simulink model "MotorXploer_1"  (R2025a)
settings: Solver=FixedStepAuto  StartTime=0.0  StopTime=inf  FixedStep=0.001  RelTol=1e-3
undefined symbols (not defined in the file or in its folder): Blocking, LF, Non
libraries: dspstat3 x4, amg_usbconverter_n_connect_lib x3, dspfdesign x1
settings Model: Creator=beamk  LastModifiedBy=tongl

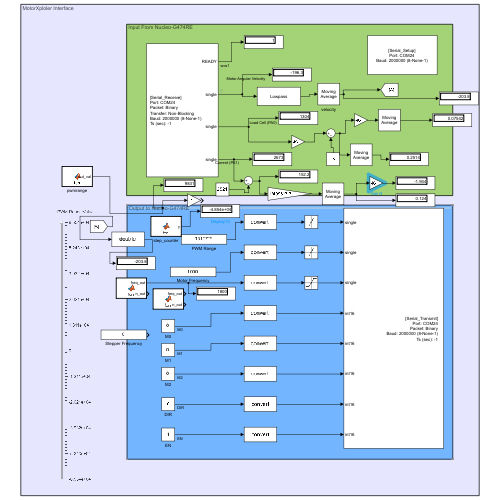
[thumbnail: Simulink's stored preview of the top-level diagram]
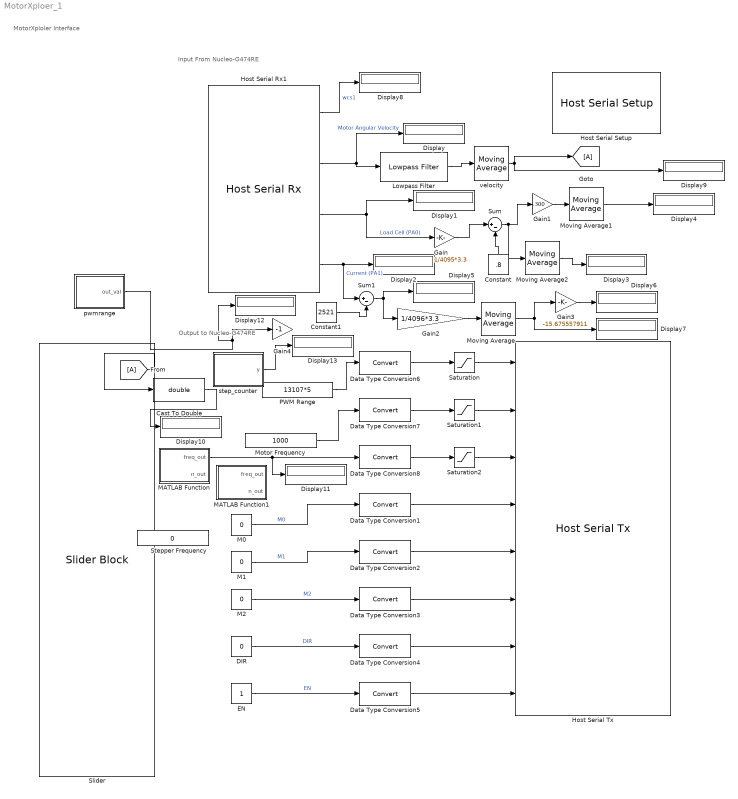
== system MotorXploer_1 ==
  note: Output to Nucleo-G474RE
  note: Input From Nucleo-G474RE
  note: MotorXploler Interface
  Cast To Double : DataTypeConversion  OutDataTypeStr=double  SaturateOnIntegerOverflow=off  RndMeth=Floor
  Constant : Constant  Value=.8
  Constant1 : Constant  Value=2521
  DIR : Constant  Value=0
  Data Type Conversion{1..8} (8 alike) : DataTypeConversion  SaturateOnIntegerOverflow=off  RndMeth=Floor
  Display{,1..13} (14 alike) : Display
  EN : Constant
  From : From
  Gain : Gain  Gain=1/4095*3.3
  Gain1 : Gain  Gain=.300
  Gain2 : Gain  Gain=1/4096*3.3
  Gain3 : Gain  Gain=-15.675557911
  Gain4 : Gain  Gain=-1
  Goto : Goto
  Host Serial Rx1 : amg_usbconverter_n_connect_lib/Host Serial Rx  conf=rx  port=<auto>  baudrate=2000000  databits=8  parity=None  stopbit=1  flowcontrol=None  transfer=Non-Blocking  timeout=5  packetmode=Binary  enableinitialvalues=off  initialvalues=[]  binheader='25'  binterminator='4E'  porttype_double=0  porttype_single=3  porttype_int8=0  porttype_uint8=0  porttype_int16=0  porttype_uint16=0  porttype_int32=0  porttype_uint32=0  asciiformat='%f,%f,%d,%d'  rx_asciiterminator="LF (0x0A - \"\\n\")"  tx_asciiterminator="CRLF (0x0D 0x0A - \"\\r\\n\")"  sampletime=-1  enablecustomportlabel=off  cinputportlabel=0  coutputportlabel=A  portpinstr=0  blockid=HostSerialRx1  inputporttype=[]  inputportwidth=[]  inputportlabel={}  outputporttype=[3 1 1 1]  outputportwidth=[1 1 1 1]  outputportlabel={'READY','single','single','single'}  compat=0  optionstring=[]  autoport='COM24'
  Host Serial Setup : amg_usbconverter_n_connect_lib/Host Serial Setup  conf=setup  port=<auto>  baudrate=2000000  databits=8  parity=None  stopbit=1  flowcontrol=None  transfer=Blocking  timeout=2  packetmode=Binary  initialvalues=[]  binheader='7E 7E'  binterminator='03 03'  porttype_double=0  porttype_single=1  porttype_int8=0  porttype_uint8=0  porttype_int16=0  porttype_uint16=0  porttype_int32=0  porttype_uint32=2  asciiformat='%d %u %x'  rx_asciiterminator="CRLF (0x0D 0x0A - \"\\r\\n\")"  tx_asciiterminator="CRLF (0x0D 0x0A - \"\\r\\n\")"  sampletime=-1  enablecustomportlabel=off  cinputportlabel=0  coutputportlabel=A  portpinstr=0  blockid=HostSerialSetup  inputporttype=[]  inputportwidth=[]  inputportlabel={}  outputporttype=[]  outputportwidth=[]  outputportlabel={}  compat=0  optionstring=[]  autoport='COM24'
  Host Serial Tx : amg_usbconverter_n_connect_lib/Host Serial Tx  conf=tx  port=<auto>  baudrate=2000000  databits=8  parity=None  stopbit=1  flowcontrol=None  transfer=Blocking  timeout=2  packetmode=Binary  initialvalues=[]  binheader='25'  binterminator='4E'  porttype_double=0  porttype_single=3  porttype_int8=0  porttype_uint8=0  porttype_int16=5  porttype_uint16=0  porttype_int32=0  porttype_uint32=0  asciiformat='%d,%f'  rx_asciiterminator="CRLF (0x0D 0x0A - \"\\r\\n\")"  tx_asciiterminator="CRLF (0x0D 0x0A - \"\\r\\n\")"  sampletime=-1  enablecustomportlabel=off  cinputportlabel=0  coutputportlabel=A  portpinstr=0  blockid=HostSerialTx  inputporttype=[1 1 1 4 4 4 4 4]  inputportwidth=[1 1 1 1 1 1 1 1]  inputportlabel={'single','single','single','int16','int16','int16','int16','int16'}  outputporttype=[]  outputportwidth=[]  outputportlabel={}  compat=0  optionstring=[]  autoport='COM24'
      settings: SourceProductName=aMG USB Converter N
  Lowpass Filter : dspfdesign/Lowpass Filter  FilterType=FIR  DesignForMinimumOrder=on  FilterOrder=50  PassbandFrequency=.6  StopbandFrequency=.7  PassbandRipple=0.1  StopbandAttenuation=80  SampleRateMode=Specify on dialog  SampleRate=100  SimulateUsing=Interpreted execution  roundingMode=Floor  coeffsDataTypeStr=fixdt(1,16)
  M0 : Constant  Value=0
  M1 : Constant  Value=0
  M2 : Constant  Value=0
  MATLAB Function : MATLAB Function  TreatAsAtomicUnit=on
  MATLAB Function1 : MATLAB Function  TreatAsAtomicUnit=on
  Motor Frequency : Constant  Value=1000  OutDataTypeStr=single
  Moving Average : dspstat3/Moving Average  Method=Sliding window  ForgettingFactorPort=off  SpecifyWindowLength=on  WindowLength=100  OverlapLength=99  AllowArbitraryInputLength=off  ForgettingFactor=0.9  SimulateUsing=Interpreted execution
  Moving Average1 : dspstat3/Moving Average  Method=Sliding window  ForgettingFactorPort=off  SpecifyWindowLength=on  WindowLength=100  OverlapLength=99  AllowArbitraryInputLength=off  ForgettingFactor=0.9  SimulateUsing=Interpreted execution
  Moving Average2 : dspstat3/Moving Average  Method=Sliding window  ForgettingFactorPort=off  SpecifyWindowLength=on  WindowLength=100  OverlapLength=99  AllowArbitraryInputLength=off  ForgettingFactor=0.9  SimulateUsing=Interpreted execution
  PWM Range : Constant  Value=13107*5  OutDataTypeStr=single
  Saturation : Saturate  UpperLimit=65535  LowerLimit=-65535
  Saturation1 : Saturate  UpperLimit=20000  LowerLimit=0
  Saturation2 : Saturate  UpperLimit=inf  LowerLimit=0
  Slider : SliderBlock  ScaleMin=-65535  ScaleMax=65535
  Stepper Frequency : Constant  Value=0  OutDataTypeStr=single
  Sum : Sum  Inputs=|+-
  Sum1 : Sum  Inputs=|+-
  pwmrange : MATLAB Function  TreatAsAtomicUnit=on
  step_counter : MATLAB Function  TreatAsAtomicUnit=on
  velocity : dspstat3/Moving Average  Method=Sliding window  ForgettingFactorPort=off  SpecifyWindowLength=on  WindowLength=4  OverlapLength=3  AllowArbitraryInputLength=off  ForgettingFactor=0.9  SimulateUsing=Interpreted execution
  wires:
  Host Serial Rx1/2 -> Lowpass Filter/1, Display/1  "Motor Angular Velocity"
  Host Serial Rx1/3 -> Gain/1, Display1/1  "Load Cell (PA0)"
  M0/1 -> Data Type Conversion1/1  "M0"
  EN/1 -> Data Type Conversion5/1  "EN"
  DIR/1 -> Data Type Conversion4/1  "DIR"
  M1/1 -> Data Type Conversion2/1  "M1"
  M2/1 -> Data Type Conversion3/1  "M2"
  Data Type Conversion1/1 -> Host Serial Tx/4
  Data Type Conversion2/1 -> Host Serial Tx/5
  Data Type Conversion3/1 -> Host Serial Tx/6
  Data Type Conversion4/1 -> Host Serial Tx/7
  Data Type Conversion5/1 -> Host Serial Tx/8
  Data Type Conversion6/1 -> Saturation/1
  Saturation/1 -> Host Serial Tx/1
  Data Type Conversion7/1 -> Saturation1/1
  Data Type Conversion8/1 -> Saturation2/1
  Saturation1/1 -> Host Serial Tx/2
  Saturation2/1 -> Host Serial Tx/3
  Host Serial Rx1/4 -> Display2/1, Sum1/1  "Current (PA1)"
  Gain/1 -> Sum/1
  Moving Average2/1 -> Display3/1
  Gain1/1 -> Moving Average1/1
  Sum/1 -> Moving Average2/1, Gain1/1
  Constant/1 -> Sum/2
  Moving Average1/1 -> Display4/1
  Constant1/1 -> Sum1/2
  Sum1/1 -> Gain2/1, Display5/1
  Gain3/1 -> Display6/1
  Moving Average/1 -> Gain3/1, Display7/1
  Gain2/1 -> Moving Average/1
  Host Serial Rx1/1 -> Display8/1  "wcs1"
  Lowpass Filter/1 -> velocity/1
  velocity/1 -> Goto/1, Display9/1
  MATLAB Function/1(freq_out) -> Data Type Conversion8/1, Display11/1
  From/1 -> Cast To Double/1
  Cast To Double/1 -> Display10/1
  pwmrange/1(out_val) -> Display12/1, Gain4/1
  step_counter/1(y) -> Display13/1
  Motor Frequency/1 -> Data Type Conversion7/1
  PWM Range/1 -> Data Type Conversion6/1

== matlab function MotorXploer_1/MATLAB Function ==
  data: freq_out output; n_out output
function [freq_out, n_out] = fcn()
%#codegen
% นี่คือฟังก์ชันที่ดัดแปลงจากตัวอย่างของคุณ
% 1. นับ sample ในตัวแปร 'count'
% 2. พอ 'count' ครบ 500 (นับ 0-499) จะเปลี่ยนความถี่
% 3. รีเซ็ต 'count' เป็น 0
% 4. ทำซ้ำจนถึง 10000 Hz

% --- 1. สร้างตัวแปร "จำค่าเก่า" (เหมือน example) ---
persistent count;
persistent freq_list;
persistent list_index;

% --- 2. กำหนดค่าเริ่มต้น (เหมือน example) ---
if isempty(count)
    count = 0; % "รีเซ็จ count เป็น 0 ใหม่"
    list_index = 1; % เริ่มที่ index แรก

    % สร้าง List ความถี่ "เริ่มต้นที่ 100hz ... จนถึง 10000hz"
    freq_list = [100:100:100000];
end

% --- 3. ส่งค่าปัจจุบันออกไปก่อน (สำคัญ!) ---
% เราส่งค่า "ปัจจุบัน" ออกไปก่อน
% แล้วค่อยอัปเดตค่าสำหรับ "รอบหน้า"
freq_out = freq_list(list_index);
n_out = count; % นี่คือตัวนับ 0, 1, 2... 499

% --- 4. โลจิกการนับ และ รีเซ็ต (เหมือน example) ---
% "เอาการ count มาใช้"
if count >= 1000  % "ถ้าครบ 500" (เพราะเรานับ 0-499 = 500 ค่า)

    % "รีเซ็จ count เป็น 0 ใหม่"
    count = 0;

    % "+ ความถี่ไป" (โดยการเลื่อน index)
    if list_index < length(freq_list) % "จนถึง 10000hz"
        list_index = list_index + 1;
    end

else
    % (ถ้ายังไม่ครบ 500)
    count = count + 1; % นับต่อไป
end

== matlab function MotorXploer_1/pwmrange ==
  data: out_val output
function out_val = fcn()
%#codegen

% --- 1. ประกาศตัวแปรจำค่า ---
persistent count;
persistent val;

% --- 2. กำหนดค่าเริ่มต้น ---
if isempty(count)
    count = 0;
    val = 0;      % เริ่มต้นที่ 0%
end

% --- 3. ส่งค่าออกไป ---
out_val = val;

% --- 4. โลจิกนับเวลา (1 วินาที) ---
% สมมติ Sample Time = 0.001s (1kHz) -> 1000 ticks = 1 วินาที
TARGET_TICKS = 5000; 

% ค่า Step 10% ของ 65535 คือ 6553.5 ปัดเป็นจำนวนเต็ม 6554
STEP_SIZE = 3277; 

if count >= TARGET_TICKS
    % === ครบ 1 วินาที ===
    count = 0; % รีเซ็ตเวลานับ
    
    % เพิ่มค่าทีละ 10%
    if val + STEP_SIZE <= 65540
        val = val + STEP_SIZE;
    else
        % ถ้าเกิน 100% (65535) ให้วนกลับไปเริ่ม 0 ใหม่
        %val = 0; 
    end
    
else
    % === ยังไม่ครบ 1 วินาที ===
    count = count + 1;
end

end

== matlab function MotorXploer_1/step_counter ==
  data: y output
function y = fcn()
%#codegen

% 1. ประกาศตัวแปร persistent เพื่อจำค่า
persistent val;      % เก็บค่าที่จะส่งออก (-65535 ถึง 65535)
persistent count;    % ตัวนับ sample เพื่อจับเวลา

% --- กำหนดจำนวน Sample ที่เท่ากับ 1 วินาที ---
% **ต้องแก้ตรงนี้ให้ตรงกับ Solver settings ของคุณ**
% ถ้า Solver Step size = 0.001 (1kHz) -> ใส่ 1000
% ถ้า Solver Step size = 0.01 (100Hz) -> ใส่ 100
samples_per_sec = 1000; 

% 2. กำหนดค่าเริ่มต้น (ทำงานครั้งแรกครั้งเดียว)
if isempty(val)
    val = -65535;    % เริ่มต้นที่ -65535
    count = 0;       % เริ่มนับที่ 0
end

% 3. ส่งค่าปัจจุบันออกไปก่อน
y = val;

% 4. โลจิกการนับเวลา (Count samples)
if count >= samples_per_sec
    % --- เมื่อนับครบ 1 วินาที (ตามค่า samples_per_sec) ---
    
    count = 0; % รีเซ็ตตัวนับ
    
    % เพิ่มค่าทีละ 1000
    next_val = val + 1000;
    
    % เช็คว่าเกิน 65535 หรือยัง
    if next_val > 65535
        val = 65535; % ตันที่ค่าสูงสุด
    else
        val = next_val; % อัปเดตค่าใหม่
    end
    
else
    % --- ถ้ายังไม่ครบ 1 วินาที ---
    count = count + 1; % นับต่อไปเรื่อยๆ
end

== matlab function MotorXploer_1/MATLAB Function1 ==
  data: freq_out output; n_out output
function [freq_out, n_out] = fcn()
%#codegen

% --- 1. ประกาศตัวแปร Persistent ---
persistent count;
persistent state;        % ตัวบอกช่วงเวลา: 1=รอเริ่ม, 2=จ่ายไฟ, 3=รอจบ
persistent current_freq; % เก็บค่าความถี่ปัจจุบันที่จะจ่ายออกไป

% --- 2. กำหนดค่าเริ่มต้น (ทำงานครั้งแรกครั้งเดียว) ---
if isempty(count)
    count = 0;
    state = 1;           % เริ่มต้นที่ช่วง "รอ 1 วิ" (State 1)
    current_freq = 100;  % เริ่มต้นที่ความถี่ 100 Hz
end

% --- 3. ส่วนควบคุมลำดับการทำงาน (State Machine) ---
% สมมติว่า Sample time คือ 1ms (1000 count = 1 วินาที)

switch state
    case 1 % === State 1: เริ่มจาก 0 รอ 1 วิ ===
        freq_out = 0;
        
        if count >= 1000 % ครบ 1 วินาที
            count = 0;   % รีเซ็ตนับ
            state = 2;   % ไปขั้นตอนต่อไป (จ่ายไฟ)
        else
            count = count + 1;
        end
        
    case 2 % === State 2: จ่ายความถี่ ค้างไว้ 3 วิ ===
        freq_out = current_freq;
        
        if count >= 3000 % ครบ 3 วินาที
            count = 0;   % รีเซ็ตนับ
            state = 3;   % ไปขั้นตอนต่อไป (กลับเป็น 0)
        else
            count = count + 1;
        end
        
    case 3 % === State 3: กลับมาเป็น 0 รอ 1 วิ ===
        freq_out = 0;
        
        if count >= 1000 % ครบ 1 วินาที (จบ 1 ลูปใหญ่)
            count = 0;   % รีเซ็ตนับ
            state = 1;   % วนกลับไปเริ่ม State 1 ใหม่
            
            % === อัปเดตค่าความถี่สำหรับรอบหน้า ===
            if current_freq < 10000
                current_freq = current_freq + 100; % เพิ่มทีละ 100
            else
                current_freq = 10000; % ตันที่ 10000 หรือจะให้วนกลับเป็น 100 ก็แก้ตรงนี้
            end
        else
            count = count + 1;
        end
        
    otherwise
        % กันเหนียว กรณี state หลุดค่า
        freq_out = 0;
        state = 1;
        count = 0;
end

% ส่งค่า count ออกไปดูเล่น (จะนับ 0 ถึง 1000 หรือ 3000 แล้วแต่ช่วง)
n_out = count;

end
